simulink model "motorPlate"  (R2019b)
settings: Solver=FixedStepAuto  StartTime=0.0  StopTime=10.0  FixedStep=0.001  RelTol=1e-3
values from neighbouring files (symbols this model uses):
  C_v = 16.5    [init.m]    (also in init2.m)
  g = 9.81    [init.m]    (also in init2.m)
  I0 = (m_p+3*m_m)*g/(3*K)    (= 0.37278)    [init.m]    (also in init2.m)
  I_p = m_p*0.04^2/12    (= 0.00012)    [init.m]    (also in init2.m)
  K = 11    [init.m]    (also in init2.m)
  m_m = 0.118    [init.m]    (also in init2.m)
  m_p = 0.9    [init.m]    (also in init2.m)
  motorPlateInit = [0;0;0;0;0;0.32]    [init.m]    (also in init2.m)
  r = 0.17    [init.m]    (also in init2.m)
undefined symbols (not defined in the file or in its folder): denc_mi, numc_mi
libraries: powerlib_meascontrol x3
settings Model: Creator=chukh  LastModifiedBy=123

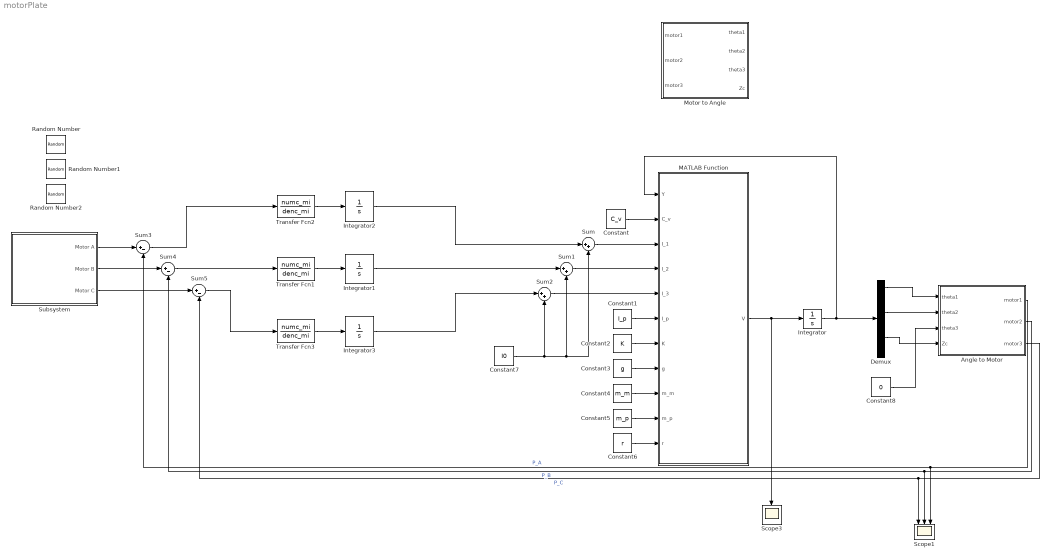
== system motorPlate ==
  Angle to Motor : MATLAB Function  TreatAsAtomicUnit=on
  Constant : Constant  Value=C_v
  Constant1 : Constant  Value=I_p
  Constant2 : Constant  Value=K
  Constant3 : Constant  Value=g
  Constant4 : Constant  Value=m_m
  Constant5 : Constant  Value=m_p
  Constant6 : Constant  Value=r
  Constant7 : Constant  Value=I0
  Constant8 : Constant  Value=0
  Demux : Demux  Outputs=6
  Integrator : Integrator  InitialCondition=motorPlateInit
  Integrator1 : Integrator  LimitOutput=on  UpperSaturationLimit=3  LowerSaturationLimit=-3
  Integrator2 : Integrator  LimitOutput=on  UpperSaturationLimit=3  LowerSaturationLimit=-3
  Integrator3 : Integrator  LimitOutput=on  UpperSaturationLimit=3  LowerSaturationLimit=-3
  MATLAB Function : MATLAB Function  TreatAsAtomicUnit=on
  Motor to Angle : MATLAB Function  TreatAsAtomicUnit=on
  Random Number : RandomNumber  Variance=0.01  Seed=13  SampleTime=0.1
  Random Number1 : RandomNumber  Variance=0.01  Seed=23  SampleTime=0.1
  Random Number2 : RandomNumber  Variance=0.01  Seed=47  SampleTime=0.1
  Scope1 : Scope  NumInputPorts=3
  Scope3 : Scope
  Subsystem : Subsystem
  Sum : Sum  Inputs=|++
  Sum1 : Sum  Inputs=|++
  Sum2 : Sum  Inputs=|++
  Sum3 : Sum  Inputs=|+-
  Sum4 : Sum  Inputs=|+-
  Sum5 : Sum  Inputs=|+-
  Transfer Fcn1 : TransferFcn  Numerator=numc_mi  Denominator=denc_mi
  Transfer Fcn2 : TransferFcn  Numerator=numc_mi  Denominator=denc_mi
  Transfer Fcn3 : TransferFcn  Numerator=numc_mi  Denominator=denc_mi
  wires:
  Constant2/1 -> MATLAB Function/7(K)
  Constant6/1 -> MATLAB Function/11(r)
  Constant3/1 -> MATLAB Function/8(g)
  Constant5/1 -> MATLAB Function/10(m_p)
  Constant1/1 -> MATLAB Function/6(I_p)
  Constant4/1 -> MATLAB Function/9(m_m)
  Constant/1 -> MATLAB Function/2(C_v)
  Integrator/1 -> Demux/1, MATLAB Function/1(Y)
  MATLAB Function/1(V) -> Scope3/1, Integrator/1
  Sum2/1 -> MATLAB Function/5(I_3)
  Sum1/1 -> MATLAB Function/4(I_2)
  Sum/1 -> MATLAB Function/3(I_1)
  Constant7/1 -> Sum/2, Sum1/2, Sum2/2
  Constant8/1 -> Angle to Motor/3(theta3)
  Demux/1 -> Angle to Motor/1(theta1)
  Demux/3 -> Angle to Motor/2(theta2)
  Subsystem/1(Motor A) -> Sum3/1
  Subsystem/2(Motor B) -> Sum4/1
  Subsystem/3(Motor C) -> Sum5/1
  Angle to Motor/3(motor3) -> Sum5/2, Scope1/1  "P_C"
  Angle to Motor/2(motor2) -> Scope1/2, Sum4/2  "P_B"
  Angle to Motor/1(motor1) -> Scope1/3, Sum3/2  "P_A"
  Transfer Fcn2/1 -> Integrator2/1
  Integrator2/1 -> Sum/1
  Sum3/1 -> Transfer Fcn2/1
  Transfer Fcn1/1 -> Integrator1/1
  Transfer Fcn3/1 -> Integrator3/1
  Sum5/1 -> Transfer Fcn3/1
  Sum4/1 -> Transfer Fcn1/1
  Integrator1/1 -> Sum1/1
  Integrator3/1 -> Sum2/1
  Demux/5 -> Angle to Motor/4(Zc)

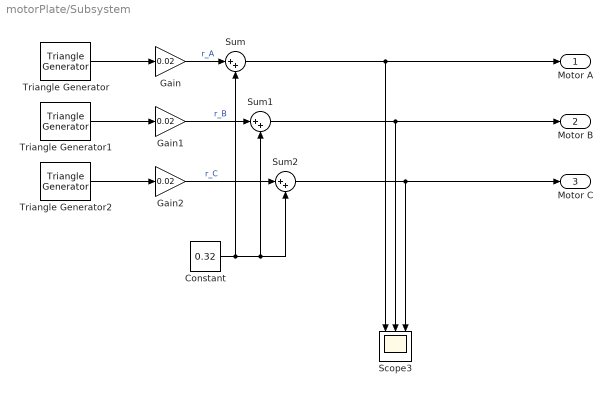
== system motorPlate/Subsystem ==
  Constant : Constant  Value=0.32
  Gain : Gain  Gain=0.02
  Gain1 : Gain  Gain=0.02
  Gain2 : Gain  Gain=0.02
  Scope3 : Scope  NumInputPorts=3
  Sum : Sum  Inputs=|++
  Sum1 : Sum  Inputs=|++
  Sum2 : Sum  Inputs=|++
  Triangle Generator : powerlib_meascontrol/Pulse & Signal Generators/Triangle Generator  Freq=0.5  Phase=90  Ts=0
      settings: SourceProductName=Simscape Electrical
  Triangle Generator1 : powerlib_meascontrol/Pulse & Signal Generators/Triangle Generator  Freq=0.5  Phase=90  Ts=0
      settings: SourceProductName=Simscape Electrical
  Triangle Generator2 : powerlib_meascontrol/Pulse & Signal Generators/Triangle Generator  Freq=0.5  Phase=90  Ts=0
      settings: SourceProductName=Simscape Electrical
  Motor A : Outport
  Motor B : Outport  Port=2
  Motor C : Outport  Port=3
  wires:
  Triangle Generator/1 -> Gain/1
  Triangle Generator1/1 -> Gain1/1
  Triangle Generator2/1 -> Gain2/1
  Gain/1 -> Sum/1  "r_A"
  Sum/1 -> Scope3/1, Motor A/1
  Constant/1 -> Sum2/2, Sum1/2, Sum/2
  Gain1/1 -> Sum1/1  "r_B"
  Gain2/1 -> Sum2/1  "r_C"
  Sum2/1 -> Motor C/1, Scope3/3
  Sum1/1 -> Motor B/1, Scope3/2

== matlab function motorPlate/Motor to Angle ==
  data: motor1 input; theta1 output; motor2 input; motor3 input; theta2 output; theta3 output; Zc output
function [theta1,theta2,theta3,Zc] = motorsToAngles(motor1, motor2, motor3)

%% Define parameters
r = 0.17;
r0B1 = [r; 0; 0];      
r0B2 = [-0.5*r; (sqrt(3)/2)*r; 0];
r0B3 = [-0.5*r; -(sqrt(3)/2)*r; 0];
r0B = [r0B1 r0B2 r0B3];
%r1C1 = r0B1; r1C2 = r0B2; r1C3 = r0B3;
r1C = r0B;

%% Find Zc
Zc = 1/3*(motor1+motor2+motor3);
r0Oc = [0;0;Zc];

%% Assemble matrices
rBC = [0 0 0; 0 0 0; motor1 motor2 motor3];
r0OC = [r0Oc r0Oc r0Oc];

%% Find A10 (Using \ operator to solve a system of linear equation since the matrix r1C is singular)
A10 = (r1C')\((rBC+r0B-r0OC)');

%% Find angles
theta2 = asin(-A10(1,3));
theta1 = asin(1/cos(theta2)*A10(2,3));
theta3 = asin(1/cos(theta2)*A10(1,2));
end

== matlab function motorPlate/MATLAB Function ==
  data: V output; Y input; C_v input; I_1 input; I_2 input; I_3 input; I_p input; K input; g input; m_m input; m_p input; r input
function V = motorPlateODE(Y,C_v,I_1,I_2,I_3,I_p,K,g,m_m,m_p,r)
%MOTORPLATEODE
%    V = MOTORPLATEODE(T,Y,C_V,I_1,I_2,I_3,I_P,K,G,M_M,M_P,R)

%    This function was generated by the Symbolic Math Toolbox version 8.4.
%    13-May-2021 20:03:52

%matrix([[theta_1f], [omega_1f], [theta_2f], [omega_2f], [dz_Cf], [z_Cf]])
t2 = I_p.^2;
t3 = Y(1);
t4 = Y(2);
t5 = Y(3);
t6 = Y(4);
t7 = Y(5);
t8 = m_m.^2;
t9 = r.^2;
t10 = r.^3;
t19 = sqrt(3.0);
t11 = t9.^2;
t12 = cos(t3);
t13 = cos(t5);
t14 = sin(t3);
t15 = sin(t5);
t16 = t2.*4.0;
t17 = t4.^2;
t18 = t6.^2;
t20 = t12.^2;
t21 = t12.^3;
t22 = t13.^2;
t23 = t13.^3;
t25 = t14.^2;
t26 = t15.^2;
t24 = t22.^2;
t27 = I_p.*m_m.*t9.*t22.*6.0;
t29 = I_p.*m_m.*t9.*t25.*t26.*6.0;
t28 = t20.*t27;
t30 = t8.*t11.*t20.*t24.*9.0;
t31 = t16+t27+t28+t29+t30;
t32 = 1.0./t31;
V = [t4;t32.*(t12.*t14.*t17.*t27+t12.*t14.*t18.*t27+t8.*t11.*t12.*t14.*t17.*t24.*9.0+t8.*t11.*t12.*t14.*t18.*t24.*9.0-C_v.*I_p.*t4.*t9.*t20.*t22.*6.0-C_v.*m_m.*t4.*t11.*t20.*t24.*9.0+I_2.*I_p.*K.*r.*t12.*t13.*t19.*2.0-I_3.*I_p.*K.*r.*t12.*t13.*t19.*2.0+I_2.*K.*m_m.*t10.*t12.*t19.*t23.*3.0-I_3.*K.*m_m.*t10.*t12.*t19.*t23.*3.0+t4.*t6.*t8.*t11.*t15.*t20.*t23.*1.8e+1+t8.*t11.*t12.*t14.*t18.*t22.*t26.*1.8e+1-t8.*t11.*t14.*t18.*t21.*t22.*t26.*9.0-t8.*t11.*t12.*t14.^3.*t18.*t22.*t26.*9.0-t4.*t6.*t8.*t11.*t13.*t15.^3.*t20.*t25.*9.0+C_v.*I_p.*t6.*t9.*t12.*t13.*t14.*t15.*6.0-I_1.*K.*m_m.*t10.*t12.*t14.*t15.*t22.*6.0+I_2.*K.*m_m.*t10.*t12.*t14.*t15.*t22.*3.0+I_3.*K.*m_m.*t10.*t12.*t14.*t15.*t22.*3.0+I_p.*m_m.*t4.*t6.*t9.*t13.*t15.*t20.*1.2e+1+t4.*t6.*t8.*t11.*t13.*t15.*t20.*t25.*9.0-t4.*t6.*t8.*t11.*t15.*t20.*t23.*t25.*9.0);t6;-r.*t32.*(I_1.*I_p.*K.*t13.*4.0-I_2.*I_p.*K.*t13.*2.0-I_3.*I_p.*K.*t13.*2.0+C_v.*I_p.*r.*t6.*t22.*6.0-t8.*t10.*t15.*t18.*t20.*t23.*1.8e+1+t8.*t10.*t15.*t18.*t20.^2.*t23.*9.0+I_2.*I_p.*K.*t14.*t15.*t19.*2.0-I_3.*I_p.*K.*t14.*t15.*t19.*2.0+C_v.*I_p.*r.*t6.*t25.*t26.*6.0+I_1.*K.*m_m.*t9.*t20.*t23.*6.0-I_2.*K.*m_m.*t9.*t20.*t23.*3.0-I_3.*K.*m_m.*t9.*t20.*t23.*3.0+C_v.*m_m.*t6.*t10.*t20.*t24.*9.0-I_p.*m_m.*r.*t13.*t15.*t18.*1.2e+1-I_p.*m_m.*r.*t4.*t6.*t12.*t14.*6.0+I_p.*m_m.*r.*t13.*t15.*t18.*t20.*6.0+I_p.*m_m.*r.*t13.*t15.*t17.*t25.*6.0+I_p.*m_m.*r.*t13.*t15.*t18.*t25.*1.2e+1-t4.*t6.*t8.*t10.*t14.*t21.*t22.*9.0+t4.*t6.*t8.*t10.*t14.*t21.*t24.*9.0+t8.*t10.*t15.*t18.*t20.*t23.*t25.*9.0-C_v.*I_p.*r.*t4.*t12.*t13.*t14.*t15.*6.0+I_p.*m_m.*r.*t4.*t6.*t12.*t14.*t22.*6.0+I_p.*m_m.*r.*t4.*t6.*t12.*t14.*t26.*1.8e+1+t4.*t6.*t8.*t10.*t14.*t21.*t22.*t26.*9.0);-(m_p+C_v.*t7.*3.0+g.*m_m.*3.0-I_1.*K-I_2.*K-I_3.*K)./(m_m.*3.0+m_p);t7];

== matlab function motorPlate/Angle to Motor ==
  data: theta1 input; motor1 output; theta2 input; theta3 input; Zc input; motor2 output; motor3 output
function [motor1, motor2, motor3] = anglesToMotors(theta1,theta2,theta3,Zc)

%% Define parameters
r = 0.17;
r0B1 = [r; 0; 0];      
r0B2 = [-0.5*r; (sqrt(3)/2)*r; 0];
r0B3 = [-0.5*r; -(sqrt(3)/2)*r; 0];
r0B = [r0B1 r0B2 r0B3];
%r1C1 = r0B1; r1C2 = r0B2; r1C3 = r0B3;
r1C = r0B;
r0Oc = [0;0;Zc];

% Find cos and sin to accelerate calculations
C1 = cos(theta1);S1 = sin(theta1);C2 = cos(theta2);S2 = sin(theta2);C3 = cos(theta3);S3 = sin(theta3);

% Rotation matrices
RotZ = [C3 S3 0; -S3 C3 0; 0 0 1];
RotY = [C2 0 -S2; 0 1 0; S2 0 C2];
RotX = [1 0 0; 0 C1 S1; 0 -S1 C1];

A10 = RotX*RotY*RotZ; A01 = A10';

% Find rCiBi (Vectors representing the motors)
rCiBi = zeros(3,3);
for i=1:3
    rCiBi(:,i) = r0Oc + A01*r1C(:,i) - r0B(:,i);
end

% Outputs to motor are the lengths of the vectors
motor1 = norm(rCiBi(:,1));
motor2 = norm(rCiBi(:,2));
motor3 = norm(rCiBi(:,3));
end
